simulink model "BTB_Case_v1"  (R2021a)
settings: Solver=FixedStepDiscrete  StartTime=0.0  StopTime=24  FixedStep=Ts_Power  RelTol=1e-3
InitFcn:
  | %Simulation parameters
  | Ts_Power = 50e-6;
  | Ts_Control = 50e-6;
  | Ts_sec = 0.05;
  | 
  | %MV Grid parameters
  | U1n = 20e3;
  | f = 50;
  | omega = 2*pi*50;
  | 
  | 
  | %LCL filter parameters
  | L_t = 100e-6;
  | C = 173e-6;
  | L_s = 100e-6;
  | R_d = 0.086;
  | R_t = omega*L_t/100;
  | R_s = omega*L_s/100;
  | 
  | %Capacitance of the DC bus
  | Cdc = 5.88e-3;
  | Rdc = 0.00001;
  | 
  | %Coupling transformers parameters
  | U2n = 400;
  | Sn1 = 3e6;
  | 
  | %Primary Subestation parameters
  | Un = 110e3;
  | Sn = 30e6;
  | 
  | %Feeder parameters
  | Le_line_1 = 12; %length km
  | R_line_1 = (0.337)*Le_line_1; %Resistance ohms
  | X_line_1 = (0.358)*Le_line_1; %Reactance ohms
  | L_line_1 = X_line_1/omega;%Inductance H
  | 
  | Le_line_2 = 10; %length km
  | R_line_2 = (0.337)*Le_line_2; %Resistance ohms
  | X_line_2 = (0.358)*Le_line_2; %Reactance ohms
  | L_line_2 = X_line_2/omega; %Inductance H
  | 
  | %PLL parameters
  | K_p_pll = 1.8;
  | K_i_pll = 1.8/0.00251;
  | 
  | %Current control loop gains
  | tau_c = 3e-3;
  | L = L_t + L_s;
  | R =R_t + R_s;
  | Kp = L/tau_c;
  | Ki = R/tau_c;
  | 
  | %DC bus voltage control loop gains
  | tau_dc = 3*tau_c;
  | 
  | %Q-V primary control loop
  | RQ = 0.15; %Q-V regulation constant
  | 
  | %24-hours household profile pu
  | ... (+21 lines)
undefined symbols (not defined in the file): D11, Delta, DiscIntNeverNeededParam, V
libraries: spsThreePhaseSeriesRLCBranchLib x16, spsThreePhaseVIMeasurementLib x13, spsRMSLib x10, simulink x6, spsSeriesRLCBranchLib x4, spsThreePhaseTransformerTwoWindingsLib x4, spsThreePhaseDynamicLoadLib x4, spsPower3phInstantaneousLib x3, eeGeneralControl x2, spsUniversalBridgeLib x2, spsVoltageMeasurementLib x2, spsThreePhaseSourceLib x1
(part 2 of 2)

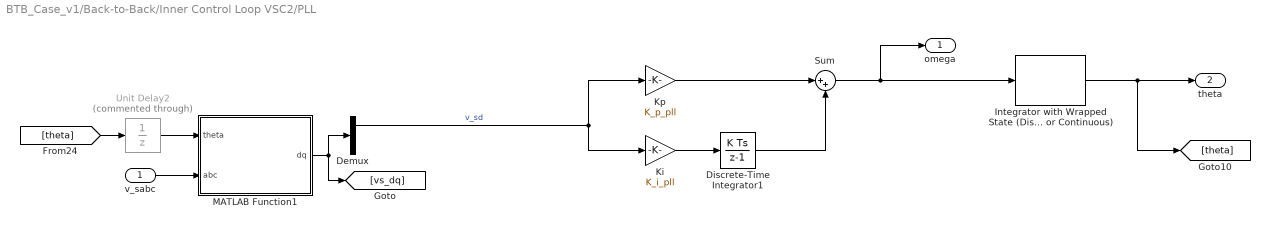
== system BTB_Case_v1/Back-to-Back/Inner Control Loop VSC2/PLL ==
  v_sabc : Inport
  Demux : Demux  Outputs=2
  Discrete-Time Integrator1 : DiscreteIntegrator  SampleTime=Ts_Control  ICPrevOutput=DiscIntNeverNeededParam  ICPrevScaledInput=DiscIntNeverNeededParam
  Integrator with Wrapped State (Discrete or Continuous) : eeGeneralControl/Integrator with Wrapped State (Discrete or Continuous)  LabelModeActiveChoice=Discrete  WrappedStateUpperValue=2*pi  WrappedStateLowerValue=0  x0=0  Ts=Ts_Control
      settings: SourceProductBaseCode=PS
  Ki : Gain  Gain=K_i_pll
  Kp : Gain  Gain=K_p_pll
  MATLAB Function1 : MATLAB Function  TreatAsAtomicUnit=on
  Sum : Sum  Inputs=|++
  Unit Delay2 : UnitDelay  Commented=through  SampleTime=Ts_Power  HasFrameUpgradeWarning=on
  omega : Outport  VectorParamsAs1DForOutWhenUnconnected=off
  theta : Outport  Port=2  VectorParamsAs1DForOutWhenUnconnected=off
  wires:
  Unit Delay2/1 -> MATLAB Function1/1(theta)
  Demux/1 -> Kp/1, Ki/1  "v_sd"
  Integrator with Wrapped State (Discrete or Continuous)/1 -> theta/1, [theta]
  Sum/1 -> Integrator with Wrapped State (Discrete or Continuous)/1, omega/1
  Discrete-Time Integrator1/1 -> Sum/2
  Kp/1 -> Sum/1
  Ki/1 -> Discrete-Time Integrator1/1
  [theta] -> Unit Delay2/1
  v_sabc/1 -> MATLAB Function1/2(abc)
  MATLAB Function1/1(dq) -> Demux/1, [vs_dq]

== matlab function BTB_Case_v1/Back-to-Back/Inner Control Loop VSC2/MATLAB Function1 ==
  data: theta input size=1; dq output; abc input
function dq  = fcn(theta,abc)
%#codegen

T_p = 2.0/3.0*[[ cos(theta), cos(theta-2.0/3.0*pi), cos(theta+2.0/3.0*pi)];
               [-sin(theta),-sin(theta-2.0/3.0*pi),-sin(theta+2.0/3.0*pi)]];
           
dq=T_p*abc;

== matlab function BTB_Case_v1/Back-to-Back/Inner Control Loop VSC2/MATLAB Function2 ==
  data: v_sdq input; i_sdq_ref output; p_ref input; q_ref input
function i_sdq_ref  = fcn(v_sdq,p_ref,q_ref)

v_sd = v_sdq(1);
v_sq = v_sdq(2);

i_sd_ref = -2/3*(p_ref*v_sd - q_ref*v_sq)/(v_sd^2+v_sq^2);
i_sq_ref = 2/3*(p_ref*v_sq - q_ref*v_sd)/(v_sd^2+v_sq^2);

i_sdq_ref=[i_sd_ref;i_sq_ref];

== matlab function BTB_Case_v1/Back-to-Back/Inner Control Loop VSC2/MATLAB Function3 ==
  data: theta input size=1; dq output; abc input
function dq  = fcn(theta,abc)
%#codegen

T_p = 2.0/3.0*[[ cos(theta), cos(theta-2.0/3.0*pi), cos(theta+2.0/3.0*pi)];
               [-sin(theta),-sin(theta-2.0/3.0*pi),-sin(theta+2.0/3.0*pi)]];
           
dq=T_p*abc;

== matlab function BTB_Case_v1/Back-to-Back/Q-V droop Controller VSC1/MATLAB Function1 ==
  data: time input; V_rms input; q_ref output; U2n parameter; Sn1 parameter; RQ parameter
function q_ref = fcn(time,V_rms,U2n,Sn1,RQ)

V_ref = 1.0; %reference voltage in p.u
V_rms_pu = V_rms/(U2n/sqrt(3));%voltage at the POI in p.u

q_ref_pu = (V_ref - V_rms_pu)*1/RQ; %Droop controller
if time<0.1
    q_ref = 0;
else
    
    q_ref = q_ref_pu*Sn1;
end

== matlab function BTB_Case_v1/Back-to-Back/Inner Control Loop VSC2/MATLAB Function5 ==
  data: theta input size=1; abc output size=3; dq input
function abc  = fcn(theta,dq)
%#codegen

T_p_inv = [[            cos(theta),            -sin(theta)];
           [ cos(theta-2.0/3.0*pi), -sin(theta-2.0/3.0*pi)];
           [ cos(theta+2.0/3.0*pi), -sin(theta+2.0/3.0*pi)]];
           
abc=T_p_inv*dq;

== matlab function BTB_Case_v1/Back-to-Back/Inner Control Loop VSC2/PLL/MATLAB Function1 ==
  data: theta input size=1; dq output; abc input
function dq  = fcn(theta,abc)
%#codegen

T_p = 2.0/3.0*[[ cos(theta), cos(theta-2.0/3.0*pi), cos(theta+2.0/3.0*pi)];
               [-sin(theta),-sin(theta-2.0/3.0*pi),-sin(theta+2.0/3.0*pi)]];
           
dq=T_p*abc;

== matlab function BTB_Case_v1/Back-to-Back/Q-V droop Controller VSC2/MATLAB Function1 ==
  data: time input; V_rms input; q_ref output; U2n parameter; Sn1 parameter; RQ parameter
function q_ref = fcn(time,V_rms,U2n,Sn1,RQ)

V_ref = 1; %reference voltage in p.u
V_rms_pu = V_rms/(U2n/sqrt(3));%voltage at the POI in p.u

q_ref_pu = (V_ref - V_rms_pu)*1/RQ; %Droop controller
if time<0.1
    q_ref = 0;
else
    
    q_ref = q_ref_pu*Sn1;
end

== matlab function BTB_Case_v1/Losses Computation ==
  data: p_fh input; p_losses output; pq_bus1 input; pq_bus2 input; pq_bus4 input; pq_bus5 input
function p_losses = fcn(p_fh,pq_bus1,pq_bus2,pq_bus4,pq_bus5)
p_bus1=pq_bus1(1); %Load Bus1
p_bus2=pq_bus2(1); %Load Bus2
p_bus4=-pq_bus4(1); %Gen Bus3
p_bus5=-pq_bus5(1); %Gen Bus4

p_losses = abs((p_fh + p_bus4 + p_bus5) - (p_bus1+p_bus2));

== matlab function BTB_Case_v1/MATLAB Function1 ==
  data: time input; p_losses input; p_ref output; p_losses_z input; p_ref_z input
function p_ref  = fcn(time,p_losses,p_losses_z,p_ref_z)

p_ref = -50e3;
tol = 10;
if time < 0.2
    p_ref = 0;
else
    if p_losses <=(p_losses_z)
        p_ref = (p_ref_z - 50e3);
    else
        p_ref = (p_ref_z);
    end
end

== matlab function BTB_Case_v1/Back-to-Back/Inner Control Loop VSC1/MATLAB Function1 ==
  data: theta input size=1; dq output; abc input
function dq  = fcn(theta,abc)
%#codegen

T_p = 2.0/3.0*[[ cos(theta), cos(theta-2.0/3.0*pi), cos(theta+2.0/3.0*pi)];
               [-sin(theta),-sin(theta-2.0/3.0*pi),-sin(theta+2.0/3.0*pi)]];
           
dq=T_p*abc;

== matlab function BTB_Case_v1/Back-to-Back/Inner Control Loop VSC1/PLL/MATLAB Function1 ==
  data: theta input size=1; dq output; abc input
function dq  = fcn(theta,abc)
%#codegen

T_p = 2.0/3.0*[[ cos(theta), cos(theta-2.0/3.0*pi), cos(theta+2.0/3.0*pi)];
               [-sin(theta),-sin(theta-2.0/3.0*pi),-sin(theta+2.0/3.0*pi)]];
           
dq=T_p*abc;

== matlab function BTB_Case_v1/Back-to-Back/Inner Control Loop VSC1/MATLAB Function ==
  data: eta_dq output; is_dq_ref input; e_dq output; vs_dq input; is_dq input; v_dc input; Kp parameter; Ki parameter; omega input; L parameter; Ts_Control parameter; e_dq_1 input; y_dq output; y_dq_1 input
function [eta_dq,e_dq,y_dq] = fcn(is_dq_ref,vs_dq,is_dq,v_dc,Kp, Ki,omega, L, Ts_Control,e_dq_1,y_dq_1)
%dq Measurements
vs_d = vs_dq(1);
vs_q = vs_dq(2);
is_d = is_dq(1);
is_q = is_dq(2);

%References
is_d_ref = is_dq_ref(1);
is_q_ref = is_dq_ref(2);

%error
e_d = is_d_ref - is_d;
e_q = is_q_ref - is_q;
e_dq = [e_d;e_q];

%Delays
y_d_1 = y_dq_1(1);
y_q_1 = y_dq_1(2);
e_d_1 = e_dq_1(1);
e_q_1 = e_dq_1(2);
%Integrator Backward Euler method
%y(n) = y(n-1) + K*[t(n) - t(n-1)]*u(n)
y_d= y_d_1 + Ki*Ts_Control*e_d;
y_q= y_q_1 + Ki*Ts_Control*e_q;

%Integrator Forward Euler method
%y(n) = y(n-1) + K*[t(n) - t(n-1)]*u(n-1)
% y_d= y_d_1 + Ki*Ts_Control*e_d_1;
% y_q= y_q_1 + Ki*Ts_Control*e_q_1;

%Integrator output
y_dq = [y_d;y_q];

%auxilary variables
u_d = Kp*e_d + y_d;
u_q = Kp*e_q + y_q;

%modulating signal computation
eta_d = 2/v_dc*(u_d -L*omega*is_q +vs_d);
eta_q = 2/v_dc*(u_q +L*omega*is_d +vs_q);

eta_dq = [eta_d;eta_q];

== matlab function BTB_Case_v1/Back-to-Back/Inner Control Loop VSC1/MATLAB Function3 ==
  data: theta input size=1; dq output; abc input
function dq  = fcn(theta,abc)
%#codegen

T_p = 2.0/3.0*[[ cos(theta), cos(theta-2.0/3.0*pi), cos(theta+2.0/3.0*pi)];
               [-sin(theta),-sin(theta-2.0/3.0*pi),-sin(theta+2.0/3.0*pi)]];
           
dq=T_p*abc;

== matlab function BTB_Case_v1/Back-to-Back/Inner Control Loop VSC1/MATLAB Function2 ==
  data: v_sdq input; i_sdq_ref output; p_ref input; q_ref input
function i_sdq_ref  = fcn(v_sdq,p_ref,q_ref)

v_sd = v_sdq(1);
v_sq = v_sdq(2);

i_sd_ref = -2/3*(p_ref*v_sd - q_ref*v_sq)/(v_sd^2+v_sq^2);
i_sq_ref = 2/3*(p_ref*v_sq - q_ref*v_sd)/(v_sd^2+v_sq^2);

i_sdq_ref=[i_sd_ref;i_sq_ref];

== matlab function BTB_Case_v1/Back-to-Back/Inner Control Loop VSC1/MATLAB Function5 ==
  data: theta input size=1; abc output size=3; dq input
function abc  = fcn(theta,dq)
%#codegen

T_p_inv = [[            cos(theta),            -sin(theta)];
           [ cos(theta-2.0/3.0*pi), -sin(theta-2.0/3.0*pi)];
           [ cos(theta+2.0/3.0*pi), -sin(theta+2.0/3.0*pi)]];
           
abc=T_p_inv*dq;

== matlab function BTB_Case_v1/Back-to-Back/Inner Control Loop VSC1/MATLAB Function4 ==
  data: time input; v_dc_ref input; p_ref output; v_dc input; y_dc_1 input; y_dc output; Cdc parameter; tau_dc parameter; Ts_Control parameter
function [p_ref,y_dc] = fcn(time,v_dc_ref,v_dc,y_dc_1, Cdc,tau_dc, Ts_Control)

error_dc = v_dc_ref^2-v_dc^2;

Kp = 2*Cdc/2/tau_dc;
Ki = 10*Kp;
y_dc = y_dc_1 + Ki*Ts_Control*error_dc;

if time<0.1
    p_ref = 0;
    y_dc = 0;
else
    p_ref = -(Kp*error_dc + y_dc);
end

== matlab function BTB_Case_v1/Back-to-Back/Inner Control Loop VSC2/MATLAB Function ==
  data: eta_dq output; is_dq_ref input; e_dq output; vs_dq input; is_dq input; v_dc input; Kp parameter; Ki parameter; omega input; L parameter; Ts_Control parameter; e_dq_1 input; y_dq output; y_dq_1 input
function [eta_dq,e_dq,y_dq] = fcn(is_dq_ref,vs_dq,is_dq,v_dc, Kp, Ki,omega,  L, Ts_Control,e_dq_1,y_dq_1)
%dq Measurements
vs_d = vs_dq(1);
vs_q = vs_dq(2);
is_d = is_dq(1);
is_q = is_dq(2);

%References
is_d_ref = is_dq_ref(1);
is_q_ref = is_dq_ref(2);

%error
e_d = is_d_ref - is_d;
e_q = is_q_ref - is_q;
e_dq = [e_d;e_q];

%Delays
y_d_1 = y_dq_1(1);
y_q_1 = y_dq_1(2);
e_d_1 = e_dq_1(1);
e_q_1 = e_dq_1(2);
%Integrator Backward Euler method
%y(n) = y(n-1) + K*[t(n) - t(n-1)]*u(n)
y_d= y_d_1 + Ki*Ts_Control*e_d;
y_q= y_q_1 + Ki*Ts_Control*e_q;

%Integrator Forward Euler method
%y(n) = y(n-1) + K*[t(n) - t(n-1)]*u(n-1)
% y_d= y_d_1 + Ki*Ts_Control*e_d_1;
% y_q= y_q_1 + Ki*Ts_Control*e_q_1;

%Integrator output
y_dq = [y_d;y_q];

%auxilary variables
u_d = Kp*e_d + y_d;
u_q = Kp*e_q + y_q;

%modulating signal computation
eta_d = 2/v_dc*(u_d -L*omega*is_q +vs_d);
eta_q = 2/v_dc*(u_q +L*omega*is_d +vs_q);

eta_dq = [eta_d;eta_q];
